simulink model "linear_model_advanced_control_project (3)"  (R2020b)
settings: Solver=VariableStepAuto  StartTime=0.0  StopTime=10  RelTol=1e-3
values from neighbouring files (symbols this model uses):
  G = -J_RH*(M_M*L/2+M*l)*(J_RH+N^2*J_m+j)*g    (= -0.22537747671)    [HighWire_Artist_Dynamic_Model.m]    (also in llllllllllllllllllll.m = -0.0465293382657; lqr_advanced_project.m = -0.0465293382657; nnnnnnnn.m = -7422.6915)
  H = -N*K_m*J_RH    (= -0.00759948)    [HighWire_Artist_Dynamic_Model.m]    (also in llllllllllllllllllll.m = -0.00486576; lqr_advanced_project.m = -0.00486576; nnnnnnnn.m = -31.5)
  K_m = 0.0109    [HighWire_Artist_Dynamic_Model.m]    (also in llllllllllllllllllll.m; lqr_advanced_project.m; nnnnnnnn.m = 21)
  L_m = 0.145    [HighWire_Artist_Dynamic_Model.m]    (also in llllllllllllllllllll.m; lqr_advanced_project.m; nnnnnnnn.m = 0.5)
  N = 14    [HighWire_Artist_Dynamic_Model.m]    (also in llllllllllllllllllll.m = 3; lqr_advanced_project.m = 0; nnnnnnnn.m = 1)
  R_m = 1.6    [HighWire_Artist_Dynamic_Model.m]    (also in llllllllllllllllllll.m; lqr_advanced_project.m; nnnnnnnn.m = 40)
  T = (M_M*L/2+M*l)*(J_RH+N^2*J_m+j)*g    (= 4.52565214276)    [HighWire_Artist_Dynamic_Model.m]    (also in llllllllllllllllllll.m = 0.312697165764; lqr_advanced_project.m = 0.312697165764; nnnnnnnn.m = 4948.461)
  W = (J_M+M*l^2)*(J_RH+N^2*J_m+j)-(J_RH)^2    (= 0.0397505665657)    [HighWire_Artist_Dynamic_Model.m]    (also in llllllllllllllllllll.m = -0.0192235420783; lqr_advanced_project.m = -0.0192235420783; nnnnnnnn.m = 60.954)
  Z = (J_M+M*l^2)*(J_RH+N^2*J_m+j)^2-J_RH^2*(J_RH+N^2*J_m+j)    (= 0.251295170273)    [HighWire_Artist_Dynamic_Model.m]    (also in llllllllllllllllllll.m = -0.00839686182665; lqr_advanced_project.m = -0.00839686182665; nnnnnnnn.m = 418.75398)
settings Model: Creator=A family  LastModifiedBy=A family

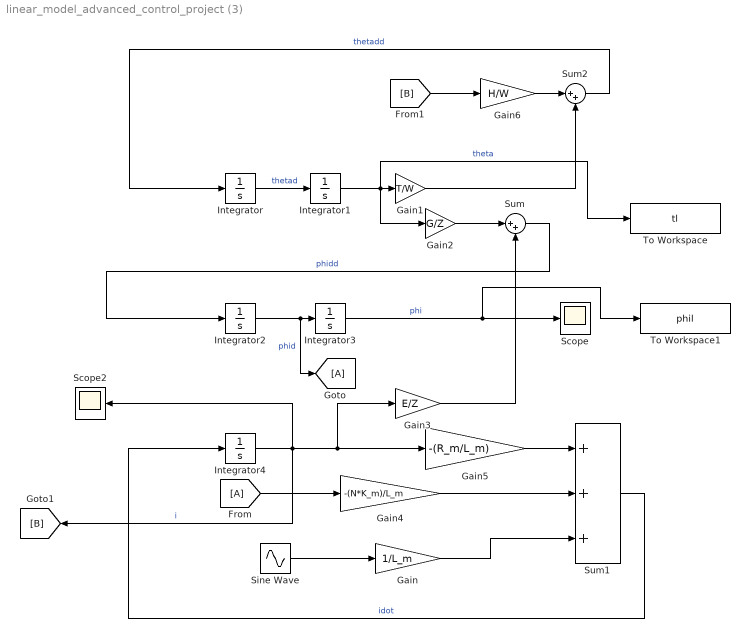
== system linear_model_advanced_control_project (3) ==
  Gain : Gain  Gain=1/L_m
  Gain1 : Gain  Gain=T/W
  Gain2 : Gain  Gain=G/Z
  Gain3 : Gain  Gain=E/Z
  Gain4 : Gain  Gain=-(N*K_m)/L_m
  Gain5 : Gain  Gain=-(R_m/L_m)
  Gain6 : Gain  Gain=H/W
  Integrator{,1..4} (5 alike) : Integrator
  Scope : Scope
  Scope2 : Scope
  Sine Wave : Sin  Amplitude=2  SampleTime=0
  Sum : Sum  Inputs=|++
  Sum1 : Sum  Inputs=+++
  Sum2 : Sum  Inputs=|++
  To Workspace : ToWorkspace  VariableName=tl  SampleTime=-1
  To Workspace1 : ToWorkspace  VariableName=phil  SampleTime=-1
  wires:
  Integrator/1 -> Integrator1/1  "thetad"
  Integrator2/1 -> [A], Integrator3/1  "phid"
  Integrator3/1 -> To Workspace1/1, Scope/1  "phi"
  Integrator1/1 -> To Workspace/1, Gain2/1, Gain1/1  "theta"
  Sum/1 -> Integrator2/1  "phidd"
  Integrator4/1 -> [B], Scope2/1, Gain5/1, Gain3/1  "i"
  Sum1/1 -> Integrator4/1  "idot"
  Gain3/1 -> Sum/2
  Gain2/1 -> Sum/1
  [A] -> Gain4/1
  Gain4/1 -> Sum1/2
  Sine Wave/1 -> Gain/1
  Gain5/1 -> Sum1/1
  Gain/1 -> Sum1/3
  [B] -> Gain6/1
  Gain6/1 -> Sum2/1
  Gain1/1 -> Sum2/2
  Sum2/1 -> Integrator/1  "thetadd"
